simulink library "my_library"  (R2025b)
settings: Solver=VariableStepAuto  StartTime=0.0  StopTime=10.0  RelTol=1e-3
undefined symbols (not defined in the file or in its folder): robot
libraries: $bdroot x13, slpidlib x3
settings Model: Creator=Junch  LastModifiedBy=Junch

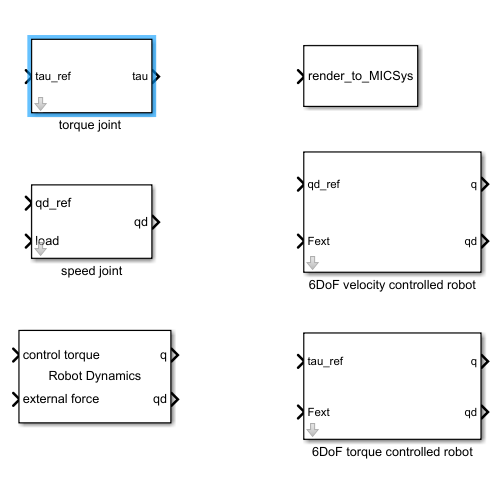
[thumbnail: Simulink's stored preview of the top-level diagram]
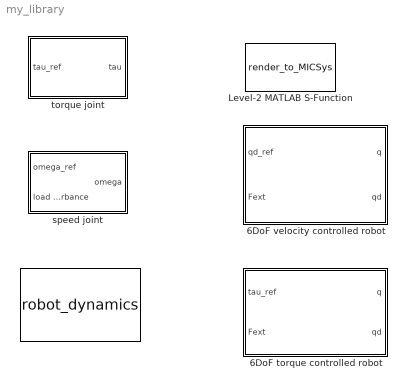
== system my_library ==
  " " : M-S-Function  FunctionName=robot_dynamics  Parameters=robot, init_pos, init_vel  mask{robot=robot, init_pos=zeros(1,robot.dof), init_vel=zeros(1,robot.dof)}
      mask prompts: init_pos "init pos:"; init_vel "init velocity:"
      mask DialogControl ParameterGroupVar Prompt: 参数
      mask Display:
      | port_label('input', 1, 'control torque')
      | port_label('input', 2, 'external force')
      | port_label('output', 1, 'q')
      | port_label('output', 2, 'qd')
      | disp('Robot Dynamics');
  6DoF torque controlled robot : Subsystem  mask{robot=robot, init_pos=zeros(1,robot.dof), b=0.1 * ones(1, robot.dof)}
      mask prompts: init_pos "init pos"; b "damping"
      mask DialogControl ParameterGroupVar Prompt: 参数
  6DoF velocity controlled robot : Subsystem  mask{q0=zeros(1,6), robot=robot}
      mask prompts: q0 "初始关节位置"; robot "机器人结构体"
      mask DialogControl ParameterGroupVar Prompt: 参数
  Level-2 MATLAB S-Function : M-S-Function  FunctionName=render_to_MICSys
  speed joint : Subsystem  mask{Jm=1e-2, bm=1e-3, gr=150, R=0.5, L=0.5e-3, K=0.125, i_kp=3.877, i_ki=3887, v_kp=15, v_ki=1.8}
      mask prompts: gr "gear ratio"; K "Ka/Kb"; i_kp "电流环增益"; i_ki "电流环积分"; v_kp "速度环增益"; v_ki "速度环积分"
      mask DialogControl ParameterGroupVar Prompt: 电机参数
      mask DialogControl Container3 Prompt: 控制参数
      mask Display:
      | port_label('output', 1, 'qd');
      | port_label('input', 1, 'qd_ref');
      | port_label('input', 2, 'load');
  "torque joint " : Subsystem  mask{Jm=1e-2, bm=1e-3, gr=150, R=0.5, L=0.5e-3, K=0.125, i_kp=3.877, i_ki=3887}
      mask prompts: gr "gear ratio"; K "Ka/Kb"; i_kp "电流环增益"; i_ki "电流环积分"
      mask DialogControl ParameterGroupVar Prompt: 电机参数
      mask DialogControl Container3 Prompt: 控制参数

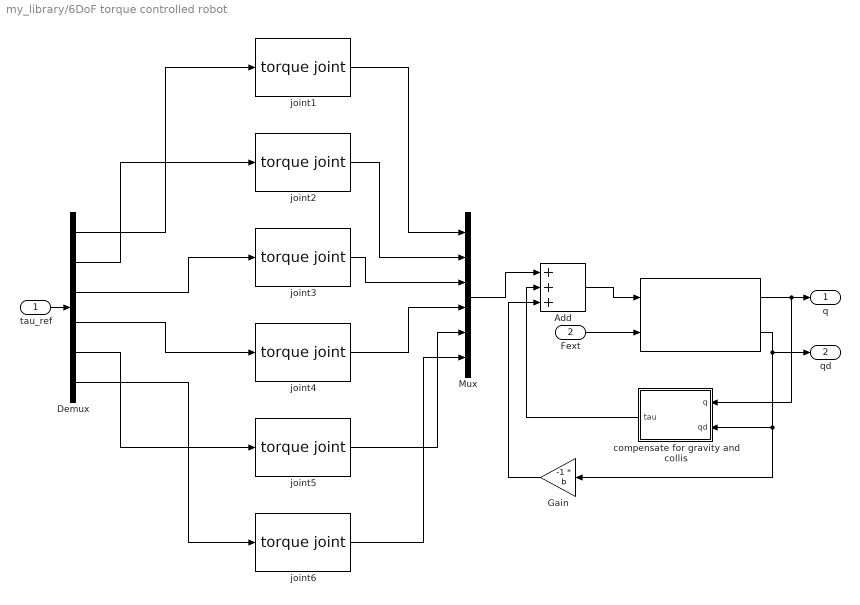
== system my_library/6DoF torque controlled robot ==
  tau_ref : Inport
  Fext : Inport  Port=2  PortDimensions=[6, robot.dof]
  " " : $bdroot/   robot=robot  init_pos=init_pos  init_vel=zeros(1,robot.dof)
  Add : Sum  Inputs=+++
  Demux : Demux  Outputs=6
  Gain : Gain  Gain=-1 * b
  Mux : Mux  Inputs=6
  compensate for gravity and collis : MATLAB Function  TreatAsAtomicUnit=on
  joint1 : $bdroot/torque joint   Jm=1e-2  bm=1e-3  gr=150  R=0.5  L=0.5e-3  K=0.125  i_kp=3.877  i_ki=3887
  joint2 : $bdroot/torque joint   Jm=1e-2  bm=1e-3  gr=150  R=0.5  L=0.5e-3  K=0.125  i_kp=3.877  i_ki=3887
  joint3 : $bdroot/torque joint   Jm=1e-2  bm=1e-3  gr=150  R=0.5  L=0.5e-3  K=0.125  i_kp=3.877  i_ki=3887
  joint4 : $bdroot/torque joint   Jm=1e-2  bm=1e-3  gr=100  R=0.5  L=0.5e-3  K=0.1  i_kp=3.877  i_ki=3887
  joint5 : $bdroot/torque joint   Jm=1e-2  bm=1e-3  gr=100  R=0.5  L=0.5e-3  K=0.09  i_kp=3.877  i_ki=3887
  joint6 : $bdroot/torque joint   Jm=1e-2  bm=1e-3  gr=100  R=0.5  L=0.5e-3  K=0.09  i_kp=3.877  i_ki=3887
  q : Outport
  qd : Outport  Port=2
  wires:
  " "/1 -> q/1, compensate for gravity and collis/1(q)
  joint5/1 -> Mux/5
  Mux/1 -> Add/1
  Demux/2 -> joint2/1
  Demux/6 -> joint6/1
  Demux/5 -> joint5/1
  Add/1 -> " "/1
  Demux/3 -> joint3/1
  Demux/1 -> joint1/1
  joint6/1 -> Mux/6
  Demux/4 -> joint4/1
  " "/2 -> qd/1, Gain/1, compensate for gravity and collis/2(qd)
  joint1/1 -> Mux/1
  joint3/1 -> Mux/3
  joint4/1 -> Mux/4
  joint2/1 -> Mux/2
  compensate for gravity and collis/1(tau) -> Add/2
  Fext/1 -> " "/2
  tau_ref/1 -> Demux/1
  Gain/1 -> Add/3

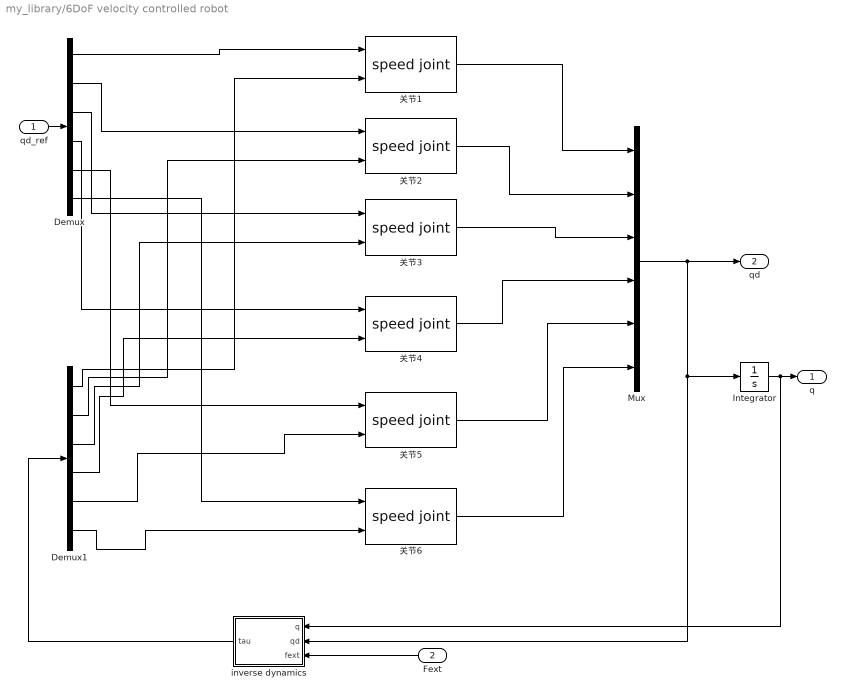
== system my_library/6DoF velocity controlled robot ==
  qd_ref : Inport
  Fext : Inport  Port=2
  Demux : Demux  Outputs=6
  Demux1 : Demux  Outputs=6
  Integrator : Integrator  InitialCondition=q0
  Mux : Mux  Inputs=6
  inverse dynamics : MATLAB Function  TreatAsAtomicUnit=on
  关节{1..6} (6 alike) : $bdroot/speed joint  Jm=1e-2  bm=1e-3  gr=150  R=0.5  L=0.5e-3  K=0.125  i_kp=3.877  i_ki=3887  v_kp=15  v_ki=1.8
  q : Outport
  qd : Outport  Port=2
  wires:
  Demux1/2 -> 关节2/2
  Mux/1 -> inverse dynamics/2(qd), Integrator/1, qd/1
  Demux1/6 -> 关节6/2
  Demux/1 -> 关节1/1
  Demux/5 -> 关节5/1
  Demux1/5 -> 关节5/2
  关节1/1 -> Mux/1
  Fext/1 -> inverse dynamics/3(fext)
  关节6/1 -> Mux/6
  Demux1/1 -> 关节1/2
  关节2/1 -> Mux/2
  Demux1/3 -> 关节3/2
  Demux/2 -> 关节2/1
  关节4/1 -> Mux/4
  Demux1/4 -> 关节4/2
  关节5/1 -> Mux/5
  关节3/1 -> Mux/3
  Demux/3 -> 关节3/1
  Demux/4 -> 关节4/1
  Demux/6 -> 关节6/1
  qd_ref/1 -> Demux/1
  Integrator/1 -> inverse dynamics/1(q), q/1
  inverse dynamics/1(tau) -> Demux1/1

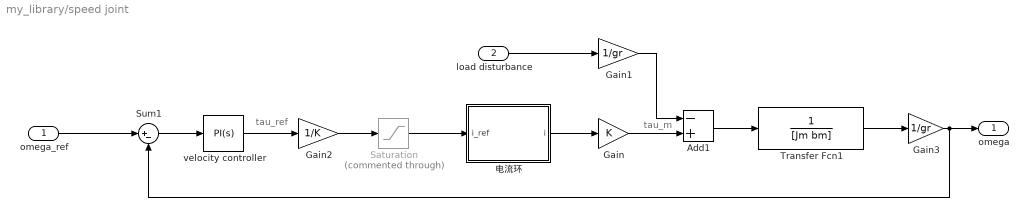
== system my_library/speed joint ==
  note: tau_ref
  note: tau_m
  omega_ref : Inport
  load disturbance : Inport  Port=2
  Add1 : Sum  Inputs=-+
  Gain : Gain  Gain=K
  Gain1 : Gain  Gain=1/gr
  Gain2 : Gain  Gain=1/K
  Gain3 : Gain  Gain=1/gr
  Saturation : Saturate  Commented=through  UpperLimit=100  LowerLimit=-100
  Sum1 : Sum  Inputs=|+-
  Transfer Fcn1 : TransferFcn  Denominator=[Jm bm]
  velocity controller : slpidlib/PID Controller  Controller=PI  Form=Parallel  TimeDomain=Continuous-time  UseExternalTs=off  SampleTime=-1  IntegratorMethod=Forward Euler  FilterMethod=Forward Euler  ControllerParametersSource=internal  P=v_kp  I=v_ki  UseKiTs=off  D=0  UseExternalDerivativeSource=off  N=100  UseFilter=on  TunerSelectOption=Transfer Function Based (PID Tuner App)  InitialConditionSource=internal  InitialConditionForIntegrator=0  InitialConditionForFilter=0  DifferentiatorICPrevScaledInput=0  ExternalReset=none  TrackingMode=off  Kt=1  LimitOutput=off  SatLimitsSource=internal  UpperSaturationLimit=inf  LowerSaturationLimit=-inf  LinearizeAsGain=on  AntiWindupMode=none  Kb=1  LimitIntegrator=off  UpperIntegratorSaturationLimit=inf  LowerIntegratorSaturationLimit=-inf  POutMin=[]  POutMax=[]  IOutMin=[]  IOutMax=[]  DOutMin=[]  DOutMax=[]  NOutMin=[]  NOutMax=[]  SumOutMin=[]  SumOutMax=[]  SaturationOutMin=[]  SaturationOutMax=[]  PParamMin=[]  PParamMax=[]  IParamMin=[]  IParamMax=[]  DParamMin=[]  DParamMax=[]  NParamMin=[]  NParamMax=[]  KbParamMin=[]  KbParamMax=[]  KtParamMin=[]  KtParamMax=[]  KbOutMin=[]  KbOutMax=[]  KtOutMin=[]  KtOutMax=[]  IntegratorOutMin=[]  IntegratorOutMax=[]  FilterOutMin=[]  FilterOutMax=[]  SumI1OutMin=[]  SumI1OutMax=[]  SumI2OutMin=[]  SumI2OutMax=[]  SumI3OutMin=[]  SumI3OutMax=[]  SumI4OutMin=[]  SumI4OutMax=[]  SumDOutMin=[]  SumDOutMax=[]  DifferentiatorOutMin=[]  DifferentiatorOutMax=[]  FilterDiffOutCoefMin=[]  FilterDiffOutCoefMax=[]  ReciprocalOutMin=[]  ReciprocalOutMax=[]  SumDenOutMin=[]  SumDenOutMax=[]  SumNumOutMin=[]  SumNumOutMax=[]  DivideOutMin=[]  DivideOutMax=[]  UdiffTsProdOutMin=[]  UdiffTsProdOutMax=[]  NTsProdOutMin=[]  NTsProdOutMax=[]  UintegralTsProdOutMin=[]  UintegralTsProdOutMax=[]  UngainTsProdOutMin=[]  UngainTsProdOutMax=[]  ClampingZeroOutDataTypeStr=Inherit: Inherit via back propagation  ClampingZeroOutMin=[]  ClampingZeroOutMax=[]  FilterDenConstantOutDataTypeStr=Inherit: Inherit via back propagation  FilterDenConstantOutMin=[]  FilterDenConstantOutMax=[]  PCopyOutDataTypeStr=Inherit: Inherit via back propagation  PCopyOutMin=[]  PCopyOutMax=[]  NCopyOutDataTypeStr=Inherit: Inherit via back propagation  NCopyOutMin=[]  NCopyOutMax=[]  IntegratorContinuousStateAttributes=''  IntegratorStateMustResolveToSignalObject=off  IntegratorRTWStateStorageClass=Auto  FilterContinuousStateAttributes=''  FilterStateMustResolveToSignalObject=off  FilterRTWStateStorageClass=Auto  ParallelPVariant=InternalParameters  IdealPVariant=Disabled  IVariant=InternalParameters  DVariant=Disabled  IntegratorVariant=Continuous  SatVariant=Disabled  AWVariant=Passthrough  PCopyVariant=Disabled  TRVariant=Disabled  FdbkBlocksVariant=Forward  IdealPFdbkVariant=Disabled  SatFdbkVariant=Disabled  DerivativeFilterVariant=Disabled  NVariant=Disabled  NCopyVariant=Disabled_SignalSpec  FilterICVariant=Disabled  IntegratorICVariant=InternalICs  ExternalResetVariant=Disabled  TRSumVariant=Passthrough  SumFdbkVariant=Disabled  SumVariant=Sum_PI  TsampFilterVariant=InternalTs  TsampNgainVariant=Passthrough  TsampIntegralVariant=Disabled_SignalSpec  ExternalSaturationOutDataTypeStr=Inherit: Same as second input  DerivativeSourceVariant=Disabled  PreIntVariant=InternalPreInt
  电流环 : Subsystem
  omega : Outport
  wires:
  Add1/1 -> Transfer Fcn1/1
  Gain2/1 -> Saturation/1
  Transfer Fcn1/1 -> Gain3/1
  Gain/1 -> Add1/2
  velocity controller/1 -> Gain2/1
  Gain1/1 -> Add1/1
  Sum1/1 -> velocity controller/1
  电流环/1(i) -> Gain/1
  load disturbance/1 -> Gain1/1
  omega_ref/1 -> Sum1/1
  Gain3/1 -> omega/1, Sum1/2
  Saturation/1 -> 电流环/1(i_ref)

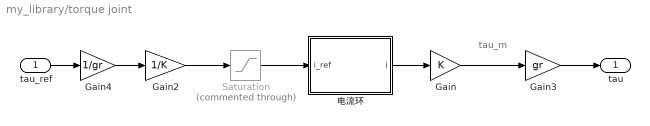
== system my_library/torque joint  ==
  note: tau_m
  tau_ref : Inport
  Gain : Gain  Gain=K
  Gain2 : Gain  Gain=1/K
  Gain3 : Gain  Gain=gr
  Gain4 : Gain  Gain=1/gr
  Saturation : Saturate  Commented=through  UpperLimit=100  LowerLimit=-100
  电流环 : Subsystem
  tau : Outport
  wires:
  Gain4/1 -> Gain2/1
  Saturation/1 -> 电流环/1(i_ref)
  Gain3/1 -> tau/1
  电流环/1(i) -> Gain/1
  tau_ref/1 -> Gain4/1
  Gain/1 -> Gain3/1
  Gain2/1 -> Saturation/1

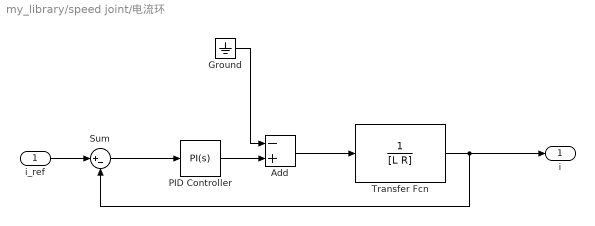
== system my_library/speed joint/电流环 ==
  i_ref : Inport
  Add : Sum  Inputs=-+
  Ground : Ground
  PID Controller : slpidlib/PID Controller  Controller=PI  Form=Parallel  TimeDomain=Continuous-time  UseExternalTs=off  SampleTime=-1  IntegratorMethod=Forward Euler  FilterMethod=Forward Euler  ControllerParametersSource=internal  P=i_kp  I=i_ki  UseKiTs=off  D=0  UseExternalDerivativeSource=off  N=100  UseFilter=on  TunerSelectOption=Transfer Function Based (PID Tuner App)  InitialConditionSource=internal  InitialConditionForIntegrator=0  InitialConditionForFilter=0  DifferentiatorICPrevScaledInput=0  ExternalReset=none  TrackingMode=off  Kt=1  LimitOutput=off  SatLimitsSource=internal  UpperSaturationLimit=inf  LowerSaturationLimit=-inf  LinearizeAsGain=on  AntiWindupMode=none  Kb=1  LimitIntegrator=off  UpperIntegratorSaturationLimit=inf  LowerIntegratorSaturationLimit=-inf  POutMin=[]  POutMax=[]  IOutMin=[]  IOutMax=[]  DOutMin=[]  DOutMax=[]  NOutMin=[]  NOutMax=[]  SumOutMin=[]  SumOutMax=[]  SaturationOutMin=[]  SaturationOutMax=[]  PParamMin=[]  PParamMax=[]  IParamMin=[]  IParamMax=[]  DParamMin=[]  DParamMax=[]  NParamMin=[]  NParamMax=[]  KbParamMin=[]  KbParamMax=[]  KtParamMin=[]  KtParamMax=[]  KbOutMin=[]  KbOutMax=[]  KtOutMin=[]  KtOutMax=[]  IntegratorOutMin=[]  IntegratorOutMax=[]  FilterOutMin=[]  FilterOutMax=[]  SumI1OutMin=[]  SumI1OutMax=[]  SumI2OutMin=[]  SumI2OutMax=[]  SumI3OutMin=[]  SumI3OutMax=[]  SumI4OutMin=[]  SumI4OutMax=[]  SumDOutMin=[]  SumDOutMax=[]  DifferentiatorOutMin=[]  DifferentiatorOutMax=[]  FilterDiffOutCoefMin=[]  FilterDiffOutCoefMax=[]  ReciprocalOutMin=[]  ReciprocalOutMax=[]  SumDenOutMin=[]  SumDenOutMax=[]  SumNumOutMin=[]  SumNumOutMax=[]  DivideOutMin=[]  DivideOutMax=[]  UdiffTsProdOutMin=[]  UdiffTsProdOutMax=[]  NTsProdOutMin=[]  NTsProdOutMax=[]  UintegralTsProdOutMin=[]  UintegralTsProdOutMax=[]  UngainTsProdOutMin=[]  UngainTsProdOutMax=[]  ClampingZeroOutDataTypeStr=Inherit: Inherit via back propagation  ClampingZeroOutMin=[]  ClampingZeroOutMax=[]  FilterDenConstantOutDataTypeStr=Inherit: Inherit via back propagation  FilterDenConstantOutMin=[]  FilterDenConstantOutMax=[]  PCopyOutDataTypeStr=Inherit: Inherit via back propagation  PCopyOutMin=[]  PCopyOutMax=[]  NCopyOutDataTypeStr=Inherit: Inherit via back propagation  NCopyOutMin=[]  NCopyOutMax=[]  IntegratorContinuousStateAttributes=''  IntegratorStateMustResolveToSignalObject=off  IntegratorRTWStateStorageClass=Auto  FilterContinuousStateAttributes=''  FilterStateMustResolveToSignalObject=off  FilterRTWStateStorageClass=Auto  ParallelPVariant=InternalParameters  IdealPVariant=Disabled  IVariant=InternalParameters  DVariant=Disabled  IntegratorVariant=Continuous  SatVariant=Disabled  AWVariant=Passthrough  PCopyVariant=Disabled  TRVariant=Disabled  FdbkBlocksVariant=Forward  IdealPFdbkVariant=Disabled  SatFdbkVariant=Disabled  DerivativeFilterVariant=Disabled  NVariant=Disabled  NCopyVariant=Disabled_SignalSpec  FilterICVariant=Disabled  IntegratorICVariant=InternalICs  ExternalResetVariant=Disabled  TRSumVariant=Passthrough  SumFdbkVariant=Disabled  SumVariant=Sum_PI  TsampFilterVariant=InternalTs  TsampNgainVariant=Passthrough  TsampIntegralVariant=Disabled_SignalSpec  ExternalSaturationOutDataTypeStr=Inherit: Same as second input  DerivativeSourceVariant=Disabled  PreIntVariant=InternalPreInt
  Sum : Sum  Inputs=|+-
  Transfer Fcn : TransferFcn  Denominator=[L R]
  i : Outport
  wires:
  Add/1 -> Transfer Fcn/1
  PID Controller/1 -> Add/2
  Sum/1 -> PID Controller/1
  i_ref/1 -> Sum/1
  Ground/1 -> Add/1
  Transfer Fcn/1 -> i/1, Sum/2

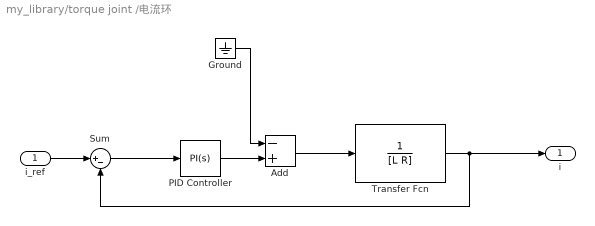
== system my_library/torque joint /电流环 ==
  i_ref : Inport
  Add : Sum  Inputs=-+
  Ground : Ground
  PID Controller : slpidlib/PID Controller  Controller=PI  Form=Parallel  TimeDomain=Continuous-time  UseExternalTs=off  SampleTime=-1  IntegratorMethod=Forward Euler  FilterMethod=Forward Euler  ControllerParametersSource=internal  P=i_kp  I=i_ki  UseKiTs=off  D=0  UseExternalDerivativeSource=off  N=100  UseFilter=on  TunerSelectOption=Transfer Function Based (PID Tuner App)  InitialConditionSource=internal  InitialConditionForIntegrator=0  InitialConditionForFilter=0  DifferentiatorICPrevScaledInput=0  ExternalReset=none  TrackingMode=off  Kt=1  LimitOutput=off  SatLimitsSource=internal  UpperSaturationLimit=inf  LowerSaturationLimit=-inf  LinearizeAsGain=on  AntiWindupMode=none  Kb=1  LimitIntegrator=off  UpperIntegratorSaturationLimit=inf  LowerIntegratorSaturationLimit=-inf  POutMin=[]  POutMax=[]  IOutMin=[]  IOutMax=[]  DOutMin=[]  DOutMax=[]  NOutMin=[]  NOutMax=[]  SumOutMin=[]  SumOutMax=[]  SaturationOutMin=[]  SaturationOutMax=[]  PParamMin=[]  PParamMax=[]  IParamMin=[]  IParamMax=[]  DParamMin=[]  DParamMax=[]  NParamMin=[]  NParamMax=[]  KbParamMin=[]  KbParamMax=[]  KtParamMin=[]  KtParamMax=[]  KbOutMin=[]  KbOutMax=[]  KtOutMin=[]  KtOutMax=[]  IntegratorOutMin=[]  IntegratorOutMax=[]  FilterOutMin=[]  FilterOutMax=[]  SumI1OutMin=[]  SumI1OutMax=[]  SumI2OutMin=[]  SumI2OutMax=[]  SumI3OutMin=[]  SumI3OutMax=[]  SumI4OutMin=[]  SumI4OutMax=[]  SumDOutMin=[]  SumDOutMax=[]  DifferentiatorOutMin=[]  DifferentiatorOutMax=[]  FilterDiffOutCoefMin=[]  FilterDiffOutCoefMax=[]  ReciprocalOutMin=[]  ReciprocalOutMax=[]  SumDenOutMin=[]  SumDenOutMax=[]  SumNumOutMin=[]  SumNumOutMax=[]  DivideOutMin=[]  DivideOutMax=[]  UdiffTsProdOutMin=[]  UdiffTsProdOutMax=[]  NTsProdOutMin=[]  NTsProdOutMax=[]  UintegralTsProdOutMin=[]  UintegralTsProdOutMax=[]  UngainTsProdOutMin=[]  UngainTsProdOutMax=[]  ClampingZeroOutDataTypeStr=Inherit: Inherit via back propagation  ClampingZeroOutMin=[]  ClampingZeroOutMax=[]  FilterDenConstantOutDataTypeStr=Inherit: Inherit via back propagation  FilterDenConstantOutMin=[]  FilterDenConstantOutMax=[]  PCopyOutDataTypeStr=Inherit: Inherit via back propagation  PCopyOutMin=[]  PCopyOutMax=[]  NCopyOutDataTypeStr=Inherit: Inherit via back propagation  NCopyOutMin=[]  NCopyOutMax=[]  IntegratorContinuousStateAttributes=''  IntegratorStateMustResolveToSignalObject=off  IntegratorRTWStateStorageClass=Auto  FilterContinuousStateAttributes=''  FilterStateMustResolveToSignalObject=off  FilterRTWStateStorageClass=Auto  ParallelPVariant=InternalParameters  IdealPVariant=Disabled  IVariant=InternalParameters  DVariant=Disabled  IntegratorVariant=Continuous  SatVariant=Disabled  AWVariant=Passthrough  PCopyVariant=Disabled  TRVariant=Disabled  FdbkBlocksVariant=Forward  IdealPFdbkVariant=Disabled  SatFdbkVariant=Disabled  DerivativeFilterVariant=Disabled  NVariant=Disabled  NCopyVariant=Disabled_SignalSpec  FilterICVariant=Disabled  IntegratorICVariant=InternalICs  ExternalResetVariant=Disabled  TRSumVariant=Passthrough  SumFdbkVariant=Disabled  SumVariant=Sum_PI  TsampFilterVariant=InternalTs  TsampNgainVariant=Passthrough  TsampIntegralVariant=Disabled_SignalSpec  ExternalSaturationOutDataTypeStr=Inherit: Same as second input  DerivativeSourceVariant=Disabled  PreIntVariant=InternalPreInt
  Sum : Sum  Inputs=|+-
  Transfer Fcn : TransferFcn  Denominator=[L R]
  i : Outport
  wires:
  Transfer Fcn/1 -> Sum/2, i/1
  Ground/1 -> Add/1
  i_ref/1 -> Sum/1
  Sum/1 -> PID Controller/1
  PID Controller/1 -> Add/2
  Add/1 -> Transfer Fcn/1

== matlab function my_library/6DoF torque controlled robot/compensate for gravity and collis ==
  data: tau output; q input; qd input; robot parameter
function tau = fcn(q, qd, robot)
tau = gravity_velocity_torque(robot, q, qd);

== matlab function my_library/6DoF velocity controlled robot/inverse dynamics ==
  data: tau output; q input; qd input; fext input size=[6, robot.dof]; robot parameter
function tau = fcn(q, qd, fext, robot)
tau = inverse_dynamics_fext(robot, q, qd, zeros(robot.dof, 1), fext);
